simulink model "skydiver"  (R2024b)
settings: Solver=VariableStepAuto  StartTime=0.0  StopTime=inf  RelTol=1e-3
settings Model: Creator=kavin  LastModifiedBy=kavin

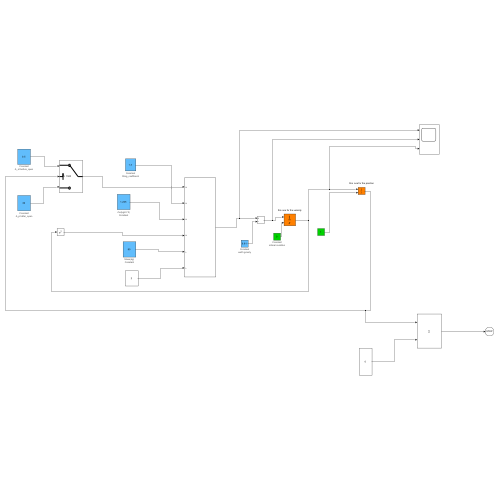
[thumbnail: Simulink's stored preview of the top-level diagram]
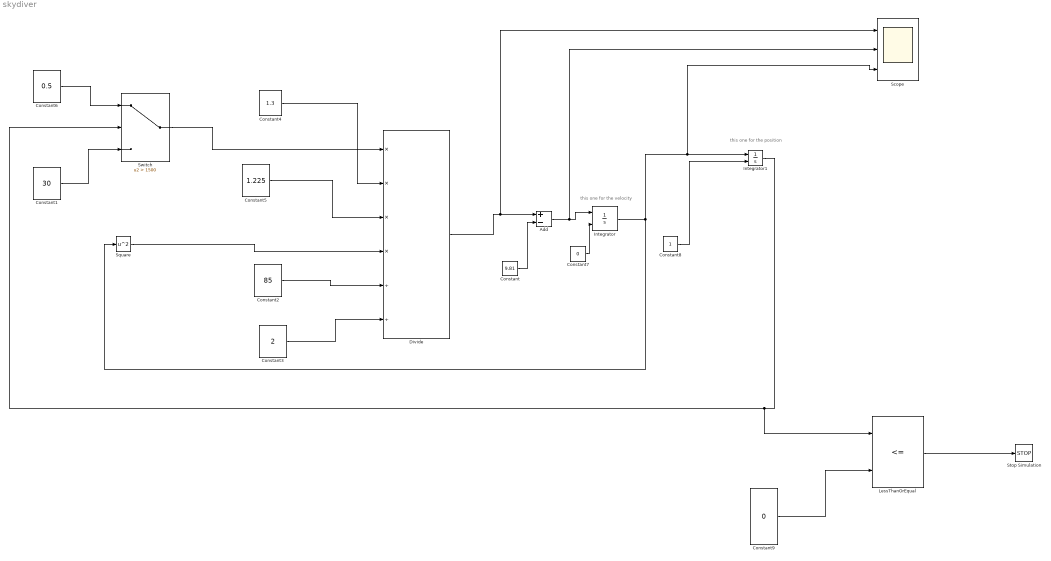
== system skydiver ==
  note: this one for the position
  note: this one for the velocity
  Add : Sum  Inputs=+-
  Constant : Constant  Value=9.81
      settings: AttributesFormatString=|
      | %<BlockType>
      | earth gravity
  Constant1 : Constant  Value=30
      settings: AttributesFormatString=|
      | %<BlockType>
      | A_p=after_open
  Constant2 : Constant  Value=85
      settings: AttributesFormatString=|
      | Mass(kg)
      | %<BlockType>
  Constant3 : Constant  Value=2
  Constant4 : Constant  Value=1.3
      settings: AttributesFormatString=|
      | %<BlockType>
      | Drag_coefficient
  Constant5 : Constant  Value=1.225
      settings: AttributesFormatString=|
      | rho(kg/m^3)
      | %<BlockType>
  Constant6 : Constant  Value=0.5
      settings: AttributesFormatString=|
      | %<BlockType>
      | A_s=before_open
  Constant7 : Constant  Value=0
      settings: AttributesFormatString=|
      | %<BlockType>
      | initinal conditon
  Constant8 : Constant
  Constant9 : Constant  Value=0
  Divide : Product  Inputs=****//
  Integrator : Integrator  InitialConditionSource=external
  Integrator1 : Integrator  InitialConditionSource=external
  LessThanOrEqual : RelationalOperator  Operator=<=  OutDataTypeStr=boolean  RndMeth=Simplest  InputSameDT=off
  Scope : Scope  NumInputPorts=3
  Square : Math  Operator=square
  Stop Simulation : Stop
  Switch : Switch  Criteria=u2 > Threshold  Threshold=1500  SaturateOnIntegerOverflow=off  InputSameDT=off
  wires:
  Constant2/1 -> Divide/5
  Constant5/1 -> Divide/3
  Divide/1 -> Scope/1, Add/1
  Constant4/1 -> Divide/2
  Switch/1 -> Divide/1
  Square/1 -> Divide/4
  Constant3/1 -> Divide/6
  Constant1/1 -> Switch/3
  Constant6/1 -> Switch/1
  Constant/1 -> Add/2
  Constant7/1 -> Integrator/2
  Constant8/1 -> Integrator1/2
  Integrator1/1 -> LessThanOrEqual/1, Switch/2
  Add/1 -> Scope/2, Integrator/1
  Integrator/1 -> Square/1, Scope/3, Integrator1/1
  Constant9/1 -> LessThanOrEqual/2
  LessThanOrEqual/1 -> Stop Simulation/1
